simulink model "missile_model_2"  (R2022b)
settings: Solver=ode4  StartTime=0.0  StopTime=10  FixedStep=0.01  RelTol=1e-3
InitFcn:
  | clc, clear, close all
  | UAV_Data
  | Sim_Parameters
values from neighbouring files (symbols this model uses):
  D = 0.150    (= 0.15)    [UAV_Data.m]    (also in UAV_Data.mat)
  I_TENSOR = [ I_xx,  0.0,  0.0 ... (first row only)    [UAV_Data.m]    (also in UAV_Data.mat = [0.084375  0  0; 0  6.5869975  0; 0  0  6.5869975])
  Init_Euler = [ 0, 0.0, 0.0 ] *  UNIT_DEG2RAD    [Sim_Parameters.m]    (also in main_Assigment3.m = [ 0.0, 0.0, 0.0 ]')
  Init_Pos = [ 0.0, 0.0, -1000.0 ]    [Sim_Parameters.m]    (also in main_Assigment3.m = [ 0.0, 0.0, -1000 ]')
  Init_Rate = [ 0, 0.0, 0.0 ] * UNIT_DEG2RAD    [Sim_Parameters.m]    (also in main_Assigment3.m = [ 0.0, 0.0, 0.0 ]')
  Init_Vel = [ 238.0, 0.0, 0.0 ]    [Sim_Parameters.m]    (also in main_Assigment3.m = [ 238, 0, 0]')
  Mass = 30.0    (= 30)    [UAV_Data.m]    (also in UAV_Data.mat)
  S = dat.S    [Assigment3_work.m]    (also in Missile_EoM.m; UAV_Data.m = 0.0176714586764; UAV_Data.mat = 0.0176714586764; verify_coeff.m)
  Theta_dot_Trim = 0.0 * UNIT_DEG2RAD    [Trim_Main_missile.m]
  Turn_dot_Trim = 0.0 * UNIT_DEG2RAD    [Trim_Main_missile.m]
  UNIT_GRAV = 9.81    [Sim_Parameters.m]
  Wn_Act = 25.0 * 2 * pi    (= 157.079632679)    [UAV_Data.m]    (also in UAV_Data.mat)
  Zeta_Act = 0.707    [UAV_Data.m]    (also in UAV_Data.mat)
libraries: aerolibconvert2 x8, simulink_extras x3, shared6dofsys x2, aerolibtransform2 x1, sharedtransform x1, sharedutil x1, aerolibatmos2 x1
settings Model: Creator=Komsun  LastModifiedBy=Komsun

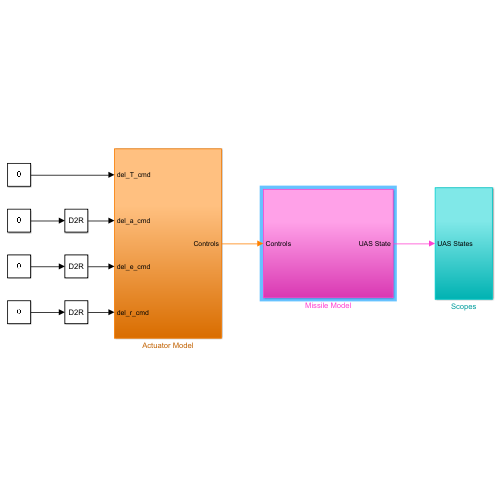
[thumbnail: Simulink's stored preview of the top-level diagram]
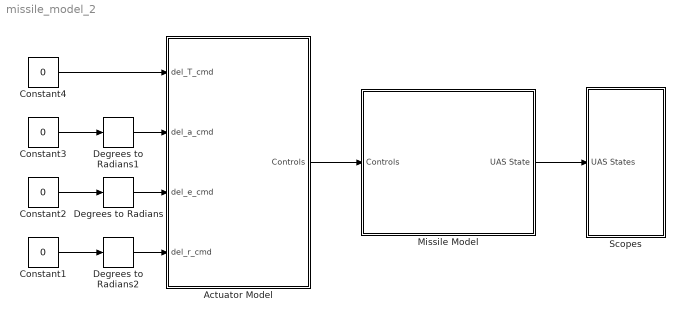
== system missile_model_2 ==
  Actuator Model : Subsystem
  Constant{1..4} (4 alike) : Constant  Value=0
  Degrees to Radians : simulink_extras/Transformations/Degrees to Radians
  Degrees to Radians1 : simulink_extras/Transformations/Degrees to Radians
  Degrees to Radians2 : simulink_extras/Transformations/Degrees to Radians
  Missile Model : Subsystem
  Scopes : Subsystem
  wires:
  Constant1/1 -> Degrees to Radians2/1
  Constant3/1 -> Degrees to Radians1/1
  Missile Model/1(UAS State) -> Scopes/1(UAS States)
  Actuator Model/1(Controls) -> Missile Model/1(Controls)
  Constant2/1 -> Degrees to Radians/1
  Constant4/1 -> Actuator Model/1(del_T_cmd)
  Degrees to Radians1/1 -> Actuator Model/2(del_a_cmd)
  Degrees to Radians/1 -> Actuator Model/3(del_e_cmd)
  Degrees to Radians2/1 -> Actuator Model/4(del_r_cmd)

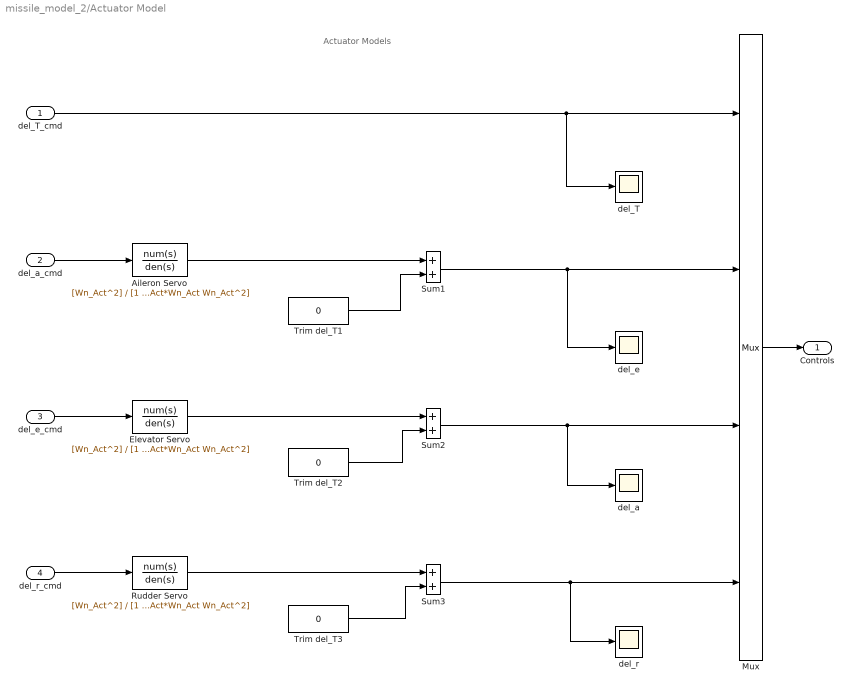
== system missile_model_2/Actuator Model ==
  note: Actuator Models
  del_T_cmd : Inport
  del_a_cmd : Inport  Port=2
  del_e_cmd : Inport  Port=3
  del_r_cmd : Inport  Port=4
  Aileron Servo : TransferFcn  Numerator=[Wn_Act^2]  Denominator=[1 2*Zeta_Act*Wn_Act Wn_Act^2]
  Elevator Servo : TransferFcn  Numerator=[Wn_Act^2]  Denominator=[1 2*Zeta_Act*Wn_Act Wn_Act^2]
  Mux : Mux
  Rudder Servo : TransferFcn  Numerator=[Wn_Act^2]  Denominator=[1 2*Zeta_Act*Wn_Act Wn_Act^2]
  Sum1 : Sum  SaturateOnIntegerOverflow=on
  Sum2 : Sum  SaturateOnIntegerOverflow=on
  Sum3 : Sum  SaturateOnIntegerOverflow=on
  Trim del_T1 : Constant  Value=0
  Trim del_T2 : Constant  Value=0
  Trim del_T3 : Constant  Value=0
  del_T : Scope
  del_a : Scope
  del_e : Scope
  del_r : Scope
  Controls : Outport
  wires:
  Mux/1 -> Controls/1
  del_T_cmd/1 -> del_T/1, Mux/1
  del_a_cmd/1 -> Aileron Servo/1
  Aileron Servo/1 -> Sum1/1
  Sum1/1 -> del_e/1, Mux/2
  Trim del_T1/1 -> Sum1/2
  Sum2/1 -> del_a/1, Mux/3
  Elevator Servo/1 -> Sum2/1
  Trim del_T2/1 -> Sum2/2
  del_e_cmd/1 -> Elevator Servo/1
  Sum3/1 -> del_r/1, Mux/4
  Trim del_T3/1 -> Sum3/2
  Rudder Servo/1 -> Sum3/1
  del_r_cmd/1 -> Rudder Servo/1

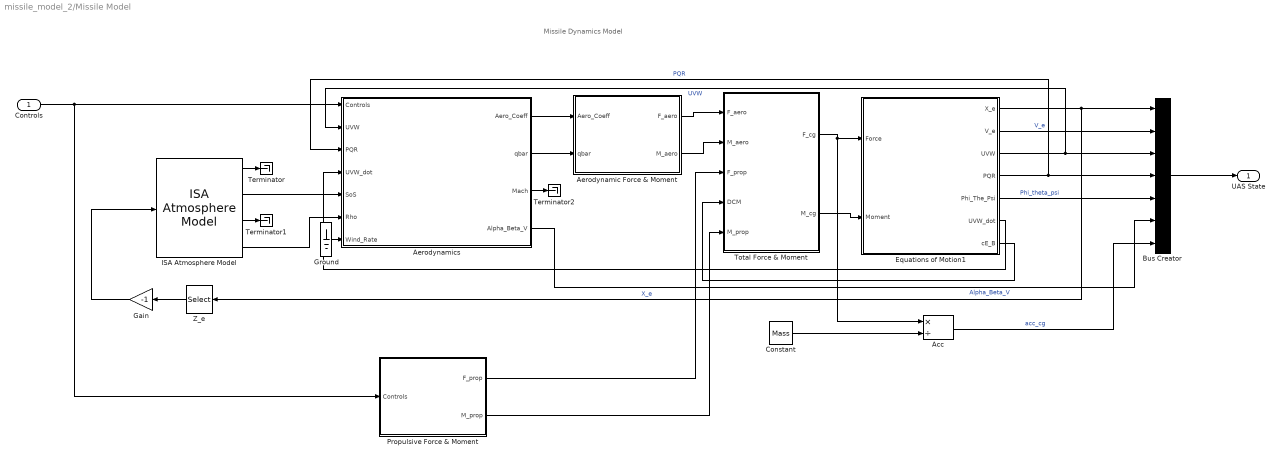
== system missile_model_2/Missile Model ==
  note: Missile Dynamics Model
  Controls : Inport
  Acc : Product  Inputs=*/  RndMeth=Zero
  Aerodynamic Force & Moment : Subsystem
  Aerodynamics : Subsystem
  Bus Creator : BusCreator  Inputs=7
  Constant : Constant  Value=Mass
  Equations of Motion1 : Subsystem
  Gain : Gain  Gain=-1
  Ground : Ground
  ISA Atmosphere Model : aerolibatmos2/ISA Atmosphere Model  custom=off  g=9.80665  gamma=1.4  R=287.0531  L=0.0065  h_trop=11000  h_strat=20000  rho0=1.225  P0=101325  T0=288.15  h0=0
  Propulsive Force & Moment : Subsystem
  Terminator : Terminator
  Terminator1 : Terminator
  Terminator2 : Terminator
  Total Force & Moment : Subsystem
  Z_e : Selector  InputPortWidth=3  IndexOptions=Index vector (dialog)  Indices=[3]  OutputSizes=1
  UAS State : Outport
  wires:
  ISA Atmosphere Model/2 -> Aerodynamics/5(SoS)
  ISA Atmosphere Model/4 -> Aerodynamics/6(Rho)
  ISA Atmosphere Model/1 -> Terminator/1
  ISA Atmosphere Model/3 -> Terminator1/1
  Aerodynamics/1(Aero_Coeff) -> Aerodynamic Force & Moment/1(Aero_Coeff)
  Aerodynamics/2(qbar) -> Aerodynamic Force & Moment/2(qbar)
  Aerodynamics/3(Mach) -> Terminator2/1
  Aerodynamic Force & Moment/1(F_aero) -> Total Force & Moment/1(F_aero)
  Aerodynamic Force & Moment/2(M_aero) -> Total Force & Moment/2(M_aero)
  Controls/1 -> Propulsive Force & Moment/1(Controls), Aerodynamics/1(Controls)
  Propulsive Force & Moment/1(F_prop) -> Total Force & Moment/3(F_prop)
  Propulsive Force & Moment/2(M_prop) -> Total Force & Moment/5(M_prop)
  Total Force & Moment/1(F_cg) -> Equations of Motion1/1(Force), Acc/1
  Total Force & Moment/2(M_cg) -> Equations of Motion1/2(Moment)
  Equations of Motion1/2(V_e) -> Bus Creator/2  "V_e"
  Constant/1 -> Acc/2
  Bus Creator/1 -> UAS State/1
  Equations of Motion1/1(X_e) -> Bus Creator/1, Z_e/1  "X_e"
  Equations of Motion1/3(UVW) -> Bus Creator/3, Aerodynamics/2(UVW)  "UVW"
  Equations of Motion1/6(UVW_dot) -> Aerodynamics/4("UVW_dot ")
  Equations of Motion1/4(PQR) -> Bus Creator/4, Aerodynamics/3(PQR)  "PQR"
  Acc/1 -> Bus Creator/7  "acc_cg"
  Aerodynamics/4(Alpha_Beta_V) -> Bus Creator/6  "Alpha_Beta_V"
  Equations of Motion1/5(Phi_The_Psi) -> Bus Creator/5  "Phi_theta_psi"
  Equations of Motion1/7(cE_B) -> Total Force & Moment/4(DCM)
  Ground/1 -> Aerodynamics/7(Wind_Rate)
  Z_e/1 -> Gain/1
  Gain/1 -> ISA Atmosphere Model/1

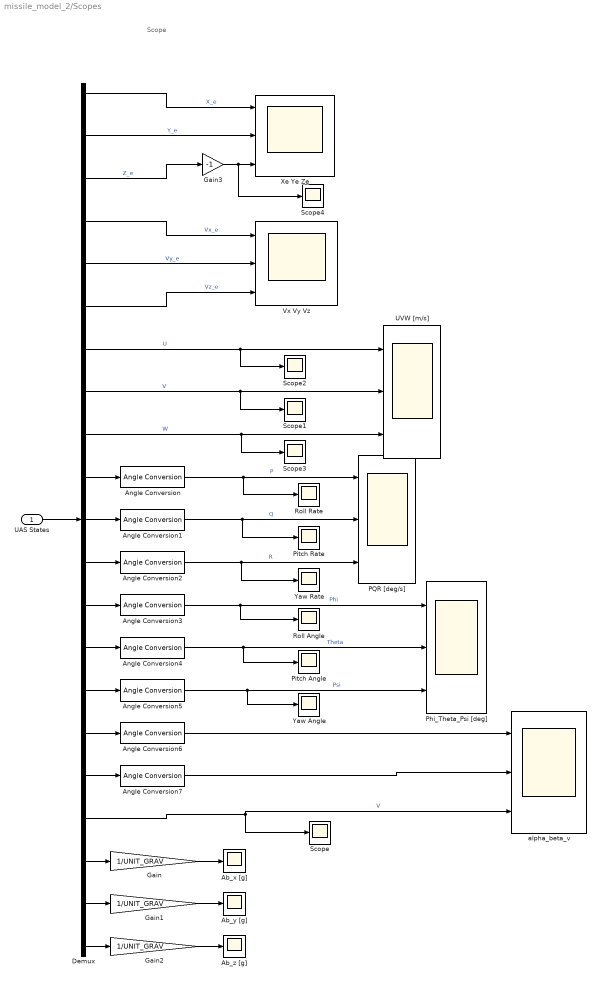
== system missile_model_2/Scopes ==
  note: Scope
  UAS States : Inport
  Ab_x [g] : Scope
  Ab_y [g] : Scope
  Ab_z [g] : Scope
  Angle Conversion{,1..7} (8 alike) : aerolibconvert2/Angle Conversion  IU=rad  OU=deg
  Demux : Demux  Outputs=21
  Gain : Gain  Gain=1/UNIT_GRAV
  Gain1 : Gain  Gain=1/UNIT_GRAV
  Gain2 : Gain  Gain=1/UNIT_GRAV
  Gain3 : Gain  Gain=-1
  PQR [deg/s] : Scope  NumInputPorts=3
  Phi_Theta_Psi [deg] : Scope  NumInputPorts=3
  Pitch Angle : Scope
  Pitch Rate : Scope
  Roll Angle : Scope
  Roll Rate : Scope
  Scope{,1..4} (5 alike) : Scope
  UVW [m/s] : Scope  NumInputPorts=3
  Vx Vy Vz : Scope  NumInputPorts=3
  Xe Ye Ze : Scope  NumInputPorts=3
  Yaw Angle : Scope
  Yaw Rate : Scope
  alpha_beta_v : Scope  NumInputPorts=3
  wires:
  UAS States/1 -> Demux/1
  Demux/1 -> Xe Ye Ze/1  "X_e"
  Demux/2 -> Xe Ye Ze/2  "Y_e"
  Demux/3 -> Gain3/1  "Z_e"
  Demux/4 -> Vx Vy Vz/1  "Vx_e"
  Demux/5 -> Vx Vy Vz/2  "Vy_e"
  Demux/6 -> Vx Vy Vz/3  "Vz_e"
  Demux/7 -> Scope2/1, UVW [m/s]/1  "U"
  Demux/8 -> Scope1/1, UVW [m/s]/2  "V"
  Demux/9 -> Scope3/1, UVW [m/s]/3  "W"
  Demux/10 -> Angle Conversion/1
  Demux/11 -> Angle Conversion1/1
  Demux/12 -> Angle Conversion2/1
  Demux/13 -> Angle Conversion3/1
  Demux/14 -> Angle Conversion4/1
  Demux/15 -> Angle Conversion5/1
  Demux/16 -> Angle Conversion6/1
  Demux/17 -> Angle Conversion7/1
  Demux/18 -> alpha_beta_v/3, Scope/1  "V"
  Demux/19 -> Gain/1
  Demux/20 -> Gain1/1
  Gain/1 -> Ab_x [g]/1
  Angle Conversion7/1 -> alpha_beta_v/2
  Angle Conversion6/1 -> alpha_beta_v/1
  Angle Conversion5/1 -> Yaw Angle/1, Phi_Theta_Psi [deg]/3  "Psi"
  Angle Conversion4/1 -> Pitch Angle/1, Phi_Theta_Psi [deg]/2  "Theta"
  Angle Conversion3/1 -> Roll Angle/1, Phi_Theta_Psi [deg]/1  "Phi"
  Angle Conversion2/1 -> PQR [deg/s]/3, Yaw Rate/1  "R"
  Angle Conversion1/1 -> Pitch Rate/1, PQR [deg/s]/2  "Q"
  Angle Conversion/1 -> Roll Rate/1, PQR [deg/s]/1  "P"
  Gain1/1 -> Ab_y [g]/1
  Demux/21 -> Gain2/1
  Gain2/1 -> Ab_z [g]/1
  Gain3/1 -> Scope4/1, Xe Ye Ze/3

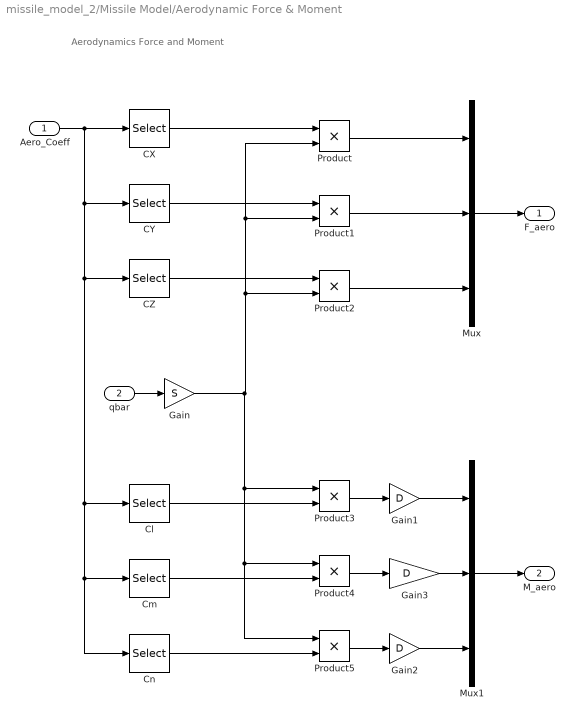
== system missile_model_2/Missile Model/Aerodynamic Force & Moment ==
  note: Aerodynamics Force and Moment
  Aero_Coeff : Inport
  qbar : Inport  Port=2
  CX : Selector  InputPortWidth=6  IndexOptions=Index vector (dialog)  Indices=[1]  OutputSizes=1
  CY : Selector  InputPortWidth=6  IndexOptions=Index vector (dialog)  Indices=[2]  OutputSizes=1
  CZ : Selector  InputPortWidth=6  IndexOptions=Index vector (dialog)  Indices=[3]  OutputSizes=1
  Cl : Selector  InputPortWidth=6  IndexOptions=Index vector (dialog)  Indices=[4]  OutputSizes=1
  Cm : Selector  InputPortWidth=6  IndexOptions=Index vector (dialog)  Indices=[5]  OutputSizes=1
  Cn : Selector  InputPortWidth=6  IndexOptions=Index vector (dialog)  Indices=[6]  OutputSizes=1
  Gain : Gain  Gain=S
  Gain1 : Gain  Gain=D
  Gain2 : Gain  Gain=D
  Gain3 : Gain  Gain=D
  Mux : Mux  Inputs=3
  Mux1 : Mux  Inputs=3
  Product{,1..5} (6 alike) : Product
  F_aero : Outport
  M_aero : Outport  Port=2
  wires:
  Aero_Coeff/1 -> Cl/1, Cn/1, Cm/1, CZ/1, CY/1, CX/1
  qbar/1 -> Gain/1
  CX/1 -> Product/1
  Gain/1 -> Product5/1, Product4/1, Product3/1, Product2/2, Product1/2, Product/2
  CY/1 -> Product1/1
  CZ/1 -> Product2/1
  Product/1 -> Mux/1
  Product1/1 -> Mux/2
  Product2/1 -> Mux/3
  Mux/1 -> F_aero/1
  Cl/1 -> Product3/2
  Cm/1 -> Product4/2
  Cn/1 -> Product5/2
  Product3/1 -> Gain1/1
  Product4/1 -> Gain3/1
  Product5/1 -> Gain2/1
  Mux1/1 -> M_aero/1
  Gain1/1 -> Mux1/1
  Gain2/1 -> Mux1/3
  Gain3/1 -> Mux1/2

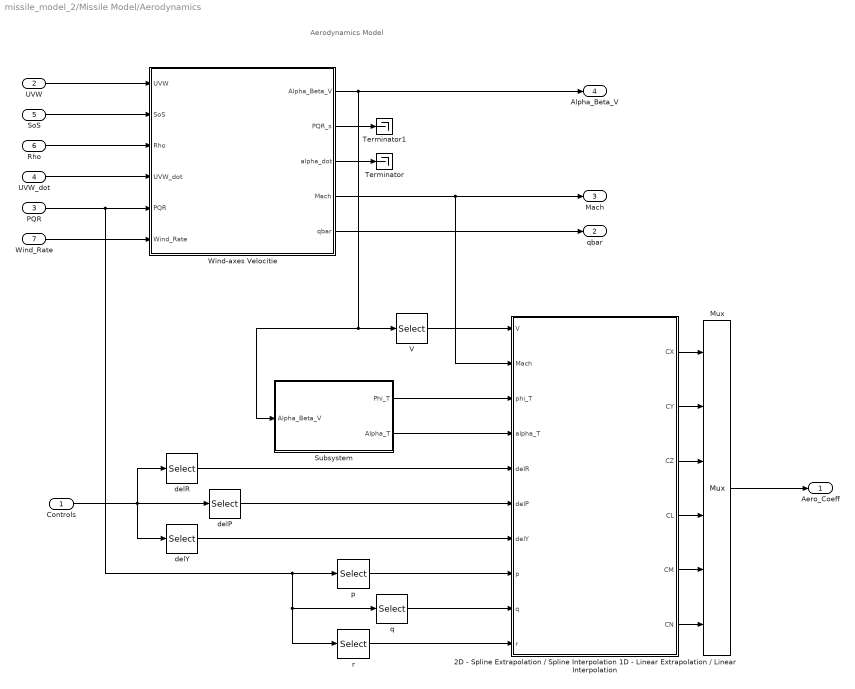
== system missile_model_2/Missile Model/Aerodynamics ==
  note: Aerodynamics Model
  Controls : Inport
  UVW : Inport  Port=2
  PQR : Inport  Port=3
  "UVW_dot " : Inport  Port=4
  SoS : Inport  Port=5
  Rho : Inport  Port=6
  Wind_Rate : Inport  Port=7
  2D - Spline Extrapolation / Spline Interpolation 1D - Linear Extrapolation / Linear Interpolation : MATLAB Function  TreatAsAtomicUnit=on
  Mux : Mux  Inputs=6
  Subsystem : Subsystem
  Terminator : Terminator
  Terminator1 : Terminator
  V : Selector  InputPortWidth=3  IndexOptions=Index vector (dialog)  Indices=[3]  OutputSizes=1
  Wind-axes Velocitie : Subsystem
  delP : Selector  InputPortWidth=4  IndexOptions=Index vector (dialog)  Indices=[3]  OutputSizes=1
  delR : Selector  InputPortWidth=4  IndexOptions=Index vector (dialog)  Indices=[2]  OutputSizes=1
  delY : Selector  InputPortWidth=4  IndexOptions=Index vector (dialog)  Indices=[4]  OutputSizes=1
  p : Selector  InputPortWidth=3  IndexOptions=Index vector (dialog)  Indices=[1]  OutputSizes=1
  q : Selector  InputPortWidth=3  IndexOptions=Index vector (dialog)  Indices=[2]  OutputSizes=1
  r : Selector  InputPortWidth=3  IndexOptions=Index vector (dialog)  Indices=[3]  OutputSizes=1
  Aero_Coeff : Outport
  qbar : Outport  Port=2
  Mach : Outport  Port=3
  Alpha_Beta_V : Outport  Port=4
  wires:
  Wind-axes Velocitie/1(Alpha_Beta_V) -> Subsystem/1(Alpha_Beta_V), V/1, Alpha_Beta_V/1
  UVW/1 -> Wind-axes Velocitie/1(UVW)
  Mux/1 -> Aero_Coeff/1
  Wind-axes Velocitie/4(Mach) -> 2D - Spline Extrapolation / Spline Interpolation 1D - Linear Extrapolation / Linear Interpolation/2(Mach), Mach/1
  Wind-axes Velocitie/5(qbar) -> qbar/1
  SoS/1 -> Wind-axes Velocitie/2(SoS)
  Rho/1 -> Wind-axes Velocitie/3(Rho)
  "UVW_dot "/1 -> Wind-axes Velocitie/4(UVW_dot)
  PQR/1 -> r/1, q/1, p/1, Wind-axes Velocitie/5(PQR)
  Wind_Rate/1 -> Wind-axes Velocitie/6(Wind_Rate)
  Wind-axes Velocitie/3(alpha_dot) -> Terminator/1
  Wind-axes Velocitie/2(PQR_s) -> Terminator1/1
  Subsystem/2(Alpha_T) -> 2D - Spline Extrapolation / Spline Interpolation 1D - Linear Extrapolation / Linear Interpolation/4(alpha_T)
  V/1 -> 2D - Spline Extrapolation / Spline Interpolation 1D - Linear Extrapolation / Linear Interpolation/1(V)
  Subsystem/1(Phi_T) -> 2D - Spline Extrapolation / Spline Interpolation 1D - Linear Extrapolation / Linear Interpolation/3(phi_T)
  Controls/1 -> delY/1, delR/1, delP/1
  delR/1 -> 2D - Spline Extrapolation / Spline Interpolation 1D - Linear Extrapolation / Linear Interpolation/5(delR)
  delP/1 -> 2D - Spline Extrapolation / Spline Interpolation 1D - Linear Extrapolation / Linear Interpolation/6(delP)
  delY/1 -> 2D - Spline Extrapolation / Spline Interpolation 1D - Linear Extrapolation / Linear Interpolation/7(delY)
  p/1 -> 2D - Spline Extrapolation / Spline Interpolation 1D - Linear Extrapolation / Linear Interpolation/8(p)
  q/1 -> 2D - Spline Extrapolation / Spline Interpolation 1D - Linear Extrapolation / Linear Interpolation/9(q)
  r/1 -> 2D - Spline Extrapolation / Spline Interpolation 1D - Linear Extrapolation / Linear Interpolation/10(r)
  2D - Spline Extrapolation / Spline Interpolation 1D - Linear Extrapolation / Linear Interpolation/1(CX) -> Mux/1
  2D - Spline Extrapolation / Spline Interpolation 1D - Linear Extrapolation / Linear Interpolation/2(CY) -> Mux/2
  2D - Spline Extrapolation / Spline Interpolation 1D - Linear Extrapolation / Linear Interpolation/3(CZ) -> Mux/3
  2D - Spline Extrapolation / Spline Interpolation 1D - Linear Extrapolation / Linear Interpolation/4(CL) -> Mux/4
  2D - Spline Extrapolation / Spline Interpolation 1D - Linear Extrapolation / Linear Interpolation/5(CM) -> Mux/5
  2D - Spline Extrapolation / Spline Interpolation 1D - Linear Extrapolation / Linear Interpolation/6(CN) -> Mux/6

== system missile_model_2/Missile Model/Equations of Motion1 ==
  note: 6DOF Motion of Equations
  Force : Inport  PortDimensions=3
  Moment : Inport  Port=2  PortDimensions=3
  Subsystem : Subsystem
  Terminator : Terminator
  X_e : Outport
  V_e : Outport  Port=2
  UVW : Outport  Port=3
  PQR : Outport  Port=4
  Phi_The_Psi : Outport  Port=5
  UVW_dot : Outport  Port=6
  cE_B : Outport  Port=7
  wires:
  Force/1 -> Subsystem/1(Forces)
  Moment/1 -> Subsystem/2(Moments)
  Subsystem/1(Ve) -> V_e/1
  Subsystem/3(Euler) -> Phi_The_Psi/1
  Subsystem/4(DCM) -> cE_B/1
  Subsystem/5(Vb) -> UVW/1
  Subsystem/6(p,q,r) -> PQR/1
  Subsystem/7(pdot,qdot,rdot) -> Terminator/1
  Subsystem/8(Ab) -> UVW_dot/1
  Subsystem/2(Xe) -> X_e/1

== system missile_model_2/Missile Model/Propulsive Force & Moment ==
  note: Propulsive Force and Moment
  Controls : Inport
  Constant : Constant  Value=0
  Mux : Mux  Inputs=3
  Mux1 : Mux  Inputs=3
  Thrust : Selector  InputPortWidth=4  IndexOptions=Index vector (dialog)  Indices=[1]  OutputSizes=1
  F_prop : Outport
  M_prop : Outport  Port=2
  wires:
  Mux1/1 -> M_prop/1
  Constant/1 -> Mux/3, Mux1/3, Mux1/2, Mux1/1, Mux/2
  Controls/1 -> Thrust/1
  Thrust/1 -> Mux/1
  Mux/1 -> F_prop/1

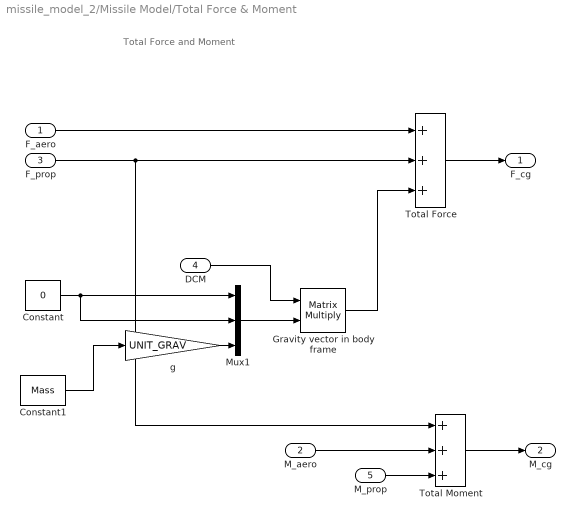
== system missile_model_2/Missile Model/Total Force & Moment ==
  note: Total Force and Moment
  F_aero : Inport  PortDimensions=3
  M_aero : Inport  Port=2  PortDimensions=3
  F_prop : Inport  Port=3  PortDimensions=3
  DCM : Inport  Port=4
  M_prop : Inport  Port=5  PortDimensions=3
  Constant : Constant  Value=0
  Constant1 : Constant  Value=Mass
  "Gravity vector in body frame " : Product  Multiplication=Matrix(*)  InputSameDT=on  SaturateOnIntegerOverflow=on  OutDataTypeStr=Inherit: Same as first input
  Mux1 : Mux  Inputs=3
  Total Force : Sum  Inputs=+++  InputSameDT=on  SaturateOnIntegerOverflow=on  OutDataTypeStr=Inherit: Same as first input
  Total Moment : Sum  Inputs=+++  InputSameDT=on  SaturateOnIntegerOverflow=on  OutDataTypeStr=Inherit: Same as first input
  g : Gain  Gain=UNIT_GRAV
  F_cg : Outport
  M_cg : Outport  Port=2
  wires:
  M_aero/1 -> Total Moment/2
  F_prop/1 -> Total Moment/1, Total Force/2
  Total Force/1 -> F_cg/1
  F_aero/1 -> Total Force/1
  M_prop/1 -> Total Moment/3
  Total Moment/1 -> M_cg/1
  Constant1/1 -> g/1
  Mux1/1 -> "Gravity vector in body frame "/2
  DCM/1 -> "Gravity vector in body frame "/1
  "Gravity vector in body frame "/1 -> Total Force/3
  Constant/1 -> Mux1/2, Mux1/1
  g/1 -> Mux1/3

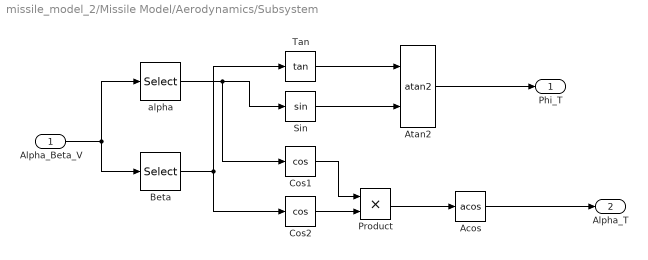
== system missile_model_2/Missile Model/Aerodynamics/Subsystem ==
  Alpha_Beta_V : Inport
  Acos : Trigonometry  Operator=acos
  Atan2 : Trigonometry  Operator=atan2
  Beta : Selector  InputPortWidth=3  IndexOptions=Index vector (dialog)  Indices=[2]  OutputSizes=1
  Cos1 : Trigonometry  Operator=cos
  Cos2 : Trigonometry  Operator=cos
  Product : Product
  Sin : Trigonometry
  Tan : Trigonometry  Operator=tan
  alpha : Selector  InputPortWidth=3  IndexOptions=Index vector (dialog)  Indices=[1]  OutputSizes=1
  Phi_T : Outport
  Alpha_T : Outport  Port=2
  wires:
  Alpha_Beta_V/1 -> alpha/1, Beta/1
  Beta/1 -> Tan/1, Cos2/1
  Tan/1 -> Atan2/1
  Sin/1 -> Atan2/2
  Atan2/1 -> Phi_T/1
  alpha/1 -> Cos1/1, Sin/1
  Cos1/1 -> Product/1
  Cos2/1 -> Product/2
  Product/1 -> Acos/1
  Acos/1 -> Alpha_T/1

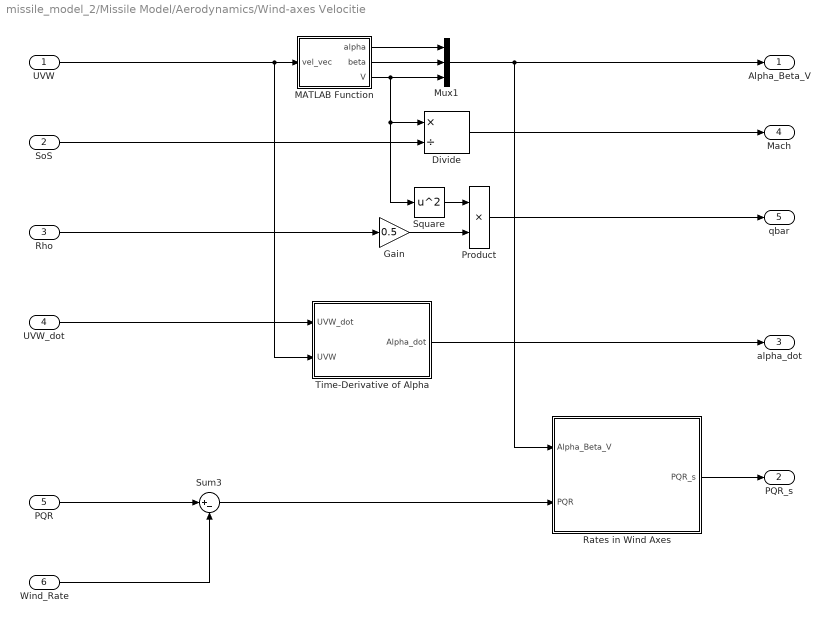
== system missile_model_2/Missile Model/Aerodynamics/Wind-axes Velocitie ==
  UVW : Inport
  SoS : Inport  Port=2
  Rho : Inport  Port=3
  UVW_dot : Inport  Port=4
  PQR : Inport  Port=5
  Wind_Rate : Inport  Port=6
  Divide : Product  Inputs=*/
  Gain : Gain  Gain=0.5
  MATLAB Function : MATLAB Function  TreatAsAtomicUnit=on
  Mux1 : Mux  Inputs=3
  Product : Product
  Rates in Wind Axes : Subsystem
  Square : Math  Operator=square
  Sum3 : Sum  Inputs=|+-  InputSameDT=on  SaturateOnIntegerOverflow=on  OutDataTypeStr=Inherit: Same as first input
  Time-Derivative of Alpha : Subsystem
  Alpha_Beta_V : Outport
  PQR_s : Outport  Port=2
  alpha_dot : Outport  Port=3
  Mach : Outport  Port=4
  qbar : Outport  Port=5
  wires:
  UVW_dot/1 -> Time-Derivative of Alpha/1(UVW_dot)
  Time-Derivative of Alpha/1(Alpha_dot) -> alpha_dot/1
  Product/1 -> qbar/1
  Rho/1 -> Gain/1
  SoS/1 -> Divide/2
  Divide/1 -> Mach/1
  Mux1/1 -> Rates in Wind Axes/1(Alpha_Beta_V), Alpha_Beta_V/1
  UVW/1 -> Time-Derivative of Alpha/2(UVW), MATLAB Function/1(vel_vec)
  MATLAB Function/1(alpha) -> Mux1/1
  MATLAB Function/2(beta) -> Mux1/2
  MATLAB Function/3(V) -> Square/1, Divide/1, Mux1/3
  Rates in Wind Axes/1(PQR_s) -> PQR_s/1
  Sum3/1 -> Rates in Wind Axes/2(PQR)
  PQR/1 -> Sum3/1
  Wind_Rate/1 -> Sum3/2
  Square/1 -> Product/1
  Gain/1 -> Product/2

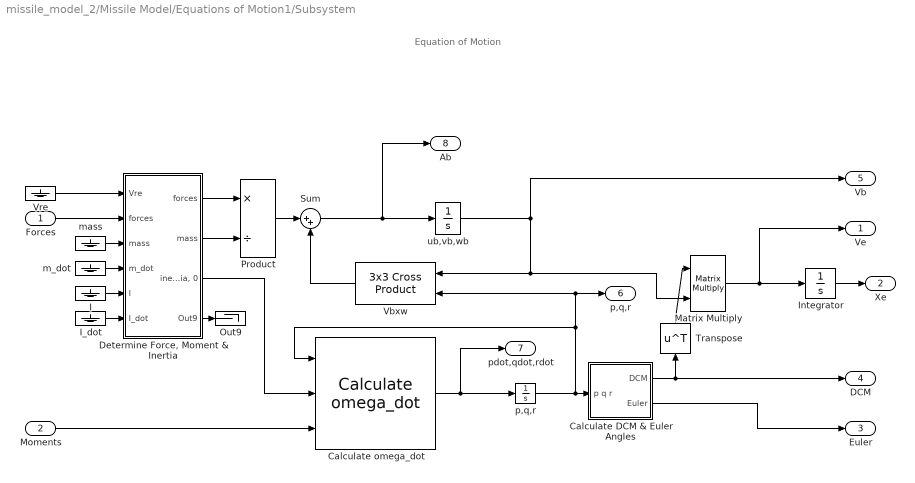
== system missile_model_2/Missile Model/Equations of Motion1/Subsystem ==
  note: Equation of Motion
  Forces : Inport  PortDimensions=3
  Moments : Inport  Port=2  PortDimensions=3
  Calculate DCM & Euler Angles : Subsystem
  Calculate omega_dot : shared6dofsys/Calculate omega_dot  aMode=aMode
  "Determine Force, Moment & Inertia" : Subsystem
  I : Ground
  I_dot : Ground
  Integrator : Integrator  InitialCondition=Init_Pos
  Matrix Multiply : Product  Multiplication=Matrix(*)
  Out9 : Terminator
  Product : Product  Inputs=*/  SaturateOnIntegerOverflow=on  OutDataTypeStr=Inherit: Same as first input
  Sum : Sum  Inputs=|++  SaturateOnIntegerOverflow=on
  Transpose : Math  Operator=transpose  SignedPower=on
  Vbxw : sharedutil/3x3 Cross Product  aMode=aMode
      settings: LibrarySourceBlock=aerolibutil/3x3 Cross Product
  Vre : Ground
  m_dot : Ground
  mass : Ground
  "p,q,r " : Integrator  InitialCondition=Init_Rate
  ub,vb,wb : Integrator  InitialCondition=Init_Vel
  Ve : Outport
  Xe : Outport  Port=2
  Euler : Outport  Port=3
  DCM : Outport  Port=4
  Vb : Outport  Port=5
  p,q,r : Outport  Port=6
  pdot,qdot,rdot : Outport  Port=7
  Ab : Outport  Port=8
  wires:
  Matrix Multiply/1 -> Integrator/1, Ve/1
  ub,vb,wb/1 -> Vb/1, Matrix Multiply/2, Vbxw/1
  Vre/1 -> "Determine Force, Moment & Inertia"/1(Vre)
  "Determine Force, Moment & Inertia"/1("forces ") -> Product/1
  I_dot/1 -> "Determine Force, Moment & Inertia"/6(I_dot)
  I/1 -> "Determine Force, Moment & Inertia"/5(I)
  Calculate omega_dot/1 -> "p,q,r "/1, pdot,qdot,rdot/1
  "Determine Force, Moment & Inertia"/4(Out9) -> Out9/1
  m_dot/1 -> "Determine Force, Moment & Inertia"/4(m_dot)
  mass/1 -> "Determine Force, Moment & Inertia"/3("mass ")
  Transpose/1 -> Matrix Multiply/1
  Calculate DCM & Euler Angles/1(DCM) -> Transpose/1, DCM/1
  Product/1 -> Sum/1
  Forces/1 -> "Determine Force, Moment & Inertia"/2(forces)
  Moments/1 -> Calculate omega_dot/3
  "p,q,r "/1 -> Calculate DCM & Euler Angles/1("p q r "), Vbxw/2, p,q,r/1, Calculate omega_dot/1
  Vbxw/1 -> Sum/2
  Calculate DCM & Euler Angles/2(Euler) -> Euler/1
  "Determine Force, Moment & Inertia"/2(mass) -> Product/2
  "Determine Force, Moment & Inertia"/3("inertia, 0") -> Calculate omega_dot/2
  Sum/1 -> Ab/1, ub,vb,wb/1
  Integrator/1 -> Xe/1

== system missile_model_2/Missile Model/Aerodynamics/Wind-axes Velocitie/Rates in Wind Axes ==
  note: Rates in Wind Axes
  Alpha_Beta_V : Inport
  PQR : Inport  Port=2
  Alpha : Selector  InputPortWidth=3  IndexOptions=Index vector (dialog)  Indices=[1]  OutputSizes=1
  Beta_Ref : Constant  Value=0
  Direction Cosine Matrix Body to Wind : aerolibtransform2/Direction Cosine Matrix Body to Wind
  Mux : Mux  Inputs=2
  transform to body axes : Product  Inputs=**  Multiplication=Matrix(*)  InputSameDT=on  SaturateOnIntegerOverflow=on  OutDataTypeStr=Inherit: Same as first input
  PQR_s : Outport
  wires:
  Alpha_Beta_V/1 -> Alpha/1
  Alpha/1 -> Mux/1
  Direction Cosine Matrix Body to Wind/1 -> transform to body axes/1  "cB_W"
  PQR/1 -> transform to body axes/2
  transform to body axes/1 -> PQR_s/1
  Mux/1 -> Direction Cosine Matrix Body to Wind/1
  Beta_Ref/1 -> Mux/2

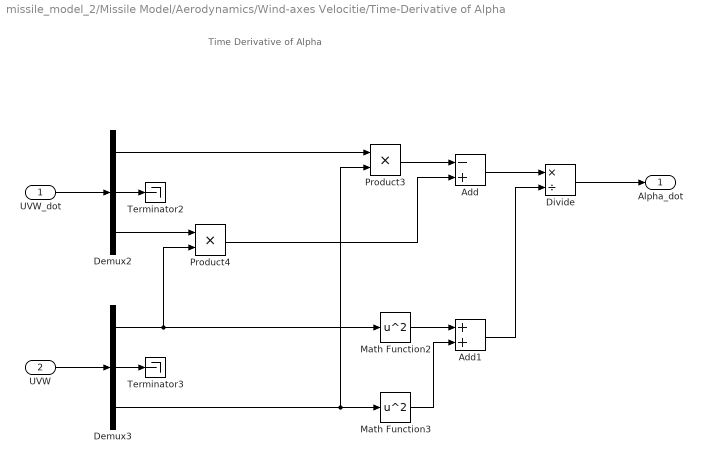
== system missile_model_2/Missile Model/Aerodynamics/Wind-axes Velocitie/Time-Derivative of Alpha ==
  note: Time Derivative of Alpha
  UVW_dot : Inport
  UVW : Inport  Port=2
  Add : Sum  Inputs=-+
  Add1 : Sum
  Demux2 : Demux  Outputs=3
  Demux3 : Demux  Outputs=3
  Divide : Product  Inputs=*/
  Math Function2 : Math  Operator=square  SignedPower=on
  Math Function3 : Math  Operator=square  SignedPower=on
  Product3 : Product
  Product4 : Product
  Terminator2 : Terminator
  Terminator3 : Terminator
  Alpha_dot : Outport
  wires:
  UVW_dot/1 -> Demux2/1
  Demux2/2 -> Terminator2/1
  Demux2/1 -> Product3/1
  UVW/1 -> Demux3/1
  Demux3/2 -> Terminator3/1
  Demux3/3 -> Math Function3/1, Product3/2
  Demux2/3 -> Product4/1
  Demux3/1 -> Math Function2/1, Product4/2
  Product4/1 -> Add/2
  Product3/1 -> Add/1
  Add/1 -> Divide/1
  Math Function2/1 -> Add1/1
  Math Function3/1 -> Add1/2
  Add1/1 -> Divide/2
  Divide/1 -> Alpha_dot/1

== system missile_model_2/Missile Model/Equations of Motion1/Subsystem/Calculate DCM & Euler Angles ==
  "p q r " : Inport
  Constant : Constant  Commented=on  Value=Theta_dot_Trim
  Constant1 : Constant  Commented=on  Value=Turn_dot_Trim
  Demux : Demux  Commented=on  Outputs=3
  Mux : Mux  Commented=on  Inputs=3
  Rotation Angles to Direction Cosine Matrix : sharedtransform/Rotation Angles to Direction Cosine Matrix  rotationOrder=ZYX  aMode=aMode
  Selector : Selector  InputPortWidth=3  IndexOptions=Index vector (dialog)  Indices=[3 2 1]  OutputSizes=1
  Sum : Sum  Commented=on  Inputs=|+-
  phi theta psi : Integrator  InitialCondition=Init_Euler
  phidot thetadot psidot : shared6dofsys/DCM & Euler Angles (Euler)/phidot thetadot psidot  SystemSampleTime=-1  VariantActivationTime=update diagram  Latency=0  AutoFrameSizeCalculation=off
  DCM : Outport
  Euler : Outport  Port=2
  wires:
  Selector/1 -> Rotation Angles to Direction Cosine Matrix/1
  phi theta psi/1 -> phidot thetadot psidot/2, Selector/1, Euler/1
  phidot thetadot psidot/1 -> phi theta psi/1
  "p q r "/1 -> phidot thetadot psidot/1
  Rotation Angles to Direction Cosine Matrix/1 -> DCM/1

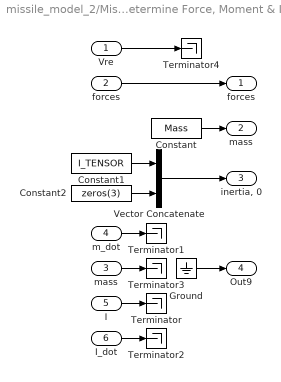
== system missile_model_2/Missile Model/Equations of Motion1/Subsystem/Determine Force, Moment & Inertia ==
  Vre : Inport
  forces : Inport  Port=2
  "mass " : Inport  Port=3
  m_dot : Inport  Port=4  OutDataTypeStr=double
  I : Inport  Port=5  OutDataTypeStr=double
  I_dot : Inport  Port=6  OutDataTypeStr=double
  Constant : Constant  Value=Mass  OutDataTypeStr=Inherit: Inherit via back propagation
  Constant1 : Constant  Value=I_TENSOR  OutDataTypeStr=Inherit: Inherit via back propagation
  Constant2 : Constant  Value=zeros(3)
  Ground : Ground
  Terminator{,1..4} (5 alike) : Terminator
  Vector Concatenate : Concatenate  Mode=Multidimensional array
  "forces " : Outport
  mass : Outport  Port=2
  "inertia, 0" : Outport  Port=3
  Out9 : Outport  Port=4
  wires:
  Vector Concatenate/1 -> "inertia, 0"/1
  Constant2/1 -> Vector Concatenate/2
  Constant1/1 -> Vector Concatenate/1
  Vre/1 -> Terminator4/1
  forces/1 -> "forces "/1
  "mass "/1 -> Terminator3/1
  I_dot/1 -> Terminator2/1
  m_dot/1 -> Terminator1/1
  I/1 -> Terminator/1
  Ground/1 -> Out9/1
  Constant/1 -> mass/1

== matlab function missile_model_2/Missile Model/Aerodynamics/Wind-axes Velocitie/MATLAB Function ==
  data: vel_vec input; alpha output; beta output; V output
function [alpha, beta, V] = calc_abv(vel_vec)

u = vel_vec(1);
v = vel_vec(2);
w = vel_vec(3);

V = norm([u v w]);          % [m/s] UAV total Speed
alpha = atan2(w,u);          % [rad] angle of attack
beta  = asin(v/V);          % [rad] sideslip angles

end

== matlab function missile_model_2/Missile Model/Aerodynamics/2D - Spline Extrapolation // Spline Interpolation 1D - Linear Extrapolation // Linear Interpolation ==
  data: V input; Mach input; CX output; phi_T input; alpha_T input; delR input; delP input; delY input; CY output; CZ output; CL output; CM output; CN output; p input; q input; r input
function [CX, CY, CZ, CL, CM, CN] = AeroCoef(V, Mach,phi_T, alpha_T, delR, delP, delY, p, q, r)

dat = load('UAV_Data.mat');
dat.Tbl_ALPHAT = dat.Tbl_ALPHAT;    % convert to rad
% alpha_T = alpha_T *180/pi;            % convert to degree

del_eff = (abs(delP) + abs(delY))/2;


B2A = rot1(-phi_T);                            % Body-to-Aeroballistics

delARPY = B2A *[delR; delP; delY];
delR_A = delARPY(1);
delP_A = delARPY(2);
delY_A = delARPY(3);

pqrA = B2A * [p; q; r];
pA = pqrA(1);
qA = pqrA(2);
rA = pqrA(3);

method = 'linear'; % 'spline', 'nearest'
method2 = 'spline';

CX_a = interp1(dat.Tbl_MACH, dat.Tbl_CX_0, Mach, method,'extrap') + interp1(dat.Tbl_MACH, dat.Tbl_CX_ALPHAT, Mach, method,'extrap')*alpha_T...
     + interp1(dat.Tbl_MACH, dat.Tbl_CX_DEL_EFF, Mach, method,'extrap')*(del_eff)^2;

CY_a = interp2(dat.Tbl_ALPHAT, dat.Tbl_MACH, dat.Tbl_CY_PHIT, alpha_T*180/pi, Mach, method2)*sin(4*phi_T)...
     + interp1(dat.Tbl_MACH, dat.Tbl_CY_DEL_Y, Mach, method,'extrap')*delY_A;

CZ_a = interp2(dat.Tbl_ALPHAT, dat.Tbl_MACH, dat.Tbl_CZ_0, alpha_T*180/pi, Mach, method2)...
     + interp2(dat.Tbl_ALPHAT, dat.Tbl_MACH, dat.Tbl_CZ_PHIT, alpha_T*180/pi, Mach, method2)*(sin(2*phi_T))^2 ...
     + interp1(dat.Tbl_MACH, dat.Tbl_CZ_DEL_P, Mach, method,'extrap')*delP_A;

CL_a = interp1(dat.Tbl_MACH, dat.Tbl_CL_ALPHAT, Mach, method,'extrap')*(alpha_T^2)*sin(4*phi_T) ...
     + interp1(dat.Tbl_MACH, dat.Tbl_CL_P, Mach, method,'extrap')*(dat.D/(2*V))*pA ...
     + interp1(dat.Tbl_MACH, dat.Tbl_CL_DEL_R, Mach, method,'extrap')*delR_A;

CM_a = interp2(dat.Tbl_ALPHAT, dat.Tbl_MACH, dat.Tbl_CM_0, alpha_T*180/pi, Mach, method2) ...
     + interp2(dat.Tbl_ALPHAT, dat.Tbl_MACH, dat.Tbl_CM_PHIT, alpha_T*180/pi, Mach, method2)*(sin(2*phi_T))^2 ...
     + interp1(dat.Tbl_MACH, dat.Tbl_CM_Q, Mach, method,'extrap')*(dat.D/(2*V))*qA ...
     + interp1(dat.Tbl_MACH, dat.Tbl_CM_DEL_P, Mach, method,'extrap')*delP_A ...
     - CZ_a*(dat.XCG - dat.XREF)/dat.D;

CN_a = interp2(dat.Tbl_ALPHAT, dat.Tbl_MACH, dat.Tbl_CN_PHIT, alpha_T*180/pi, Mach, method2)*sin(4*phi_T)...
     + interp1(dat.Tbl_MACH, dat.Tbl_CN_R, Mach, method,'extrap')*(dat.D/(2*V))*rA ...
     + interp1(dat.Tbl_MACH, dat.Tbl_CN_DEL_Y, Mach, method,'extrap')*delY_A ...
     + CY_a*(dat.XCG - dat.XREF)/dat.D;

%% Aerodynamics Coefficients in body coordinate
CXYZ = B2A.' * [CX_a; CY_a; CZ_a];
CX = CXYZ(1);
CY = CXYZ(2);
CZ = CXYZ(3);

CLMN = B2A.' * [CL_a; CM_a; CN_a];
CL = CLMN(1);
CM = CLMN(2);
CN = CLMN(3);

function out = rot1(x)
    out = [1 0 0; 0 cos(x) sin(x); 0 -sin(x) cos(x)];
end

end
